simulink model "ANN_project"  (R2019b)
settings: Solver=ode45  StartTime=0.0  StopTime=0.6  RelTol=1e-3  EnableMultiTasking=on
libraries: powerlib x20
settings Model: Creator=Administrator  LastModifiedBy=Dell
settings DataIOCC: LimitDataPoints=on  SaveFormat=Array  SignalLoggingSaveFormat=ModelDataLogs  ReturnWorkspaceOutputs=off
settings OptimizationCC: ExpressionDepthLimit=2147483647  LifeSpan=inf
settings DebuggingCC: UnderspecifiedInitializationDetection=Classic  MergeDetectMultiDrivingBlocksExec=none  SolverPrmCheckMsg=warning  FcnCallInpInsideContextMsg=warning  StateNameClashWarn=warning  SFUnexpectedBacktrackingDiag=warning  SFNoUnconditionalDefaultTransitionDiag=warning  SFExecutionAtInitializationDiag=none  ArithmeticOperatorsInVariantConditions=warning
settings HardwareCC: ProdBitPerPointer=32  ProdBitPerSizeT=32  ProdBitPerPtrDiffT=32  ProdLargestAtomicFloat=None  ProdIntDivRoundTo=Undefined  ProdEndianess=Unspecified  ProdWordSize=32  ProdHWDeviceType=32-bit Generic
settings ModelReferenceCC: PropagateSignalLabelsOutOfModel=off
settings SFSimCC: SimUseLocalCustomCode=off  CustomCodeUndefinedFunction=UseInterfaceOnly
settings RTWCC: RTWUseLocalCustomCode=off
settings CodeAppCC: StateflowObjectComments=on
settings GRTTargetCC: TargetLangStandard=C89/C90 (ANSI)  GeneratePreprocessorConditionals=Disable all  CombineOutputUpdateFcns=off  GRTInterface=on
settings ConfigComp: CovMetricSettings=dw  CovHtmlReporting=on  CovSaveCumulativeToWorkspaceVar=on  CovSaveSingleToWorkspaceVar=on  CovExternalEMLEnable=off  CovSFcnEnable=off
settings SimscapeCC: SimscapeNormalizeSystem=off

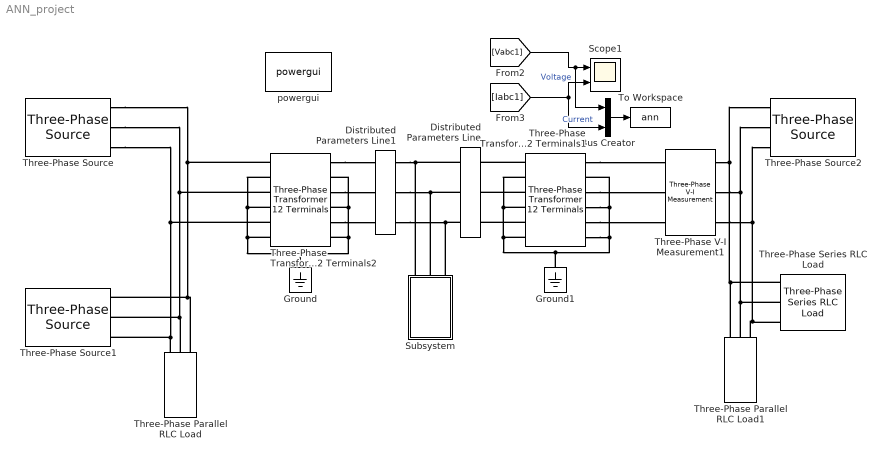
== system ANN_project ==
  Bus Creator : BusCreator  Inputs=2
  Distributed Parameters Line : powerlib/Elements/Distributed Parameters Line  Phases=3  Frequency=50  Resistance=[0.0132 0.132]  Inductance="[0.9337e-3  4.1264e-3]"  Capacitance=[12.74e-9 7.751e-9]  Length=33  x1=[-0.0002 1.11094093111666e-09 0 0;-0.00015 1.10646242430815e-09 15635.779124401 -78733.8101924462;-0.0001 1.10171091445278e-09 16870.5471169946 -78478.5008535489;-5e-05 1.09668757391454e-09 18101.1525545264 -78203.828118865]  x2=[-0.0002 1.10664892847414e-09 0 0;-0.00015 1.10142238341835e-09 15586.3909292958 -78738.689788468;-0.0001 1.0959240788704e-09 16821.2416601515 -78484.1556036391;-5e-05 1.09015537145464e-09 18051.9420013292 -78210.2566277985]  x3=[-0.0002 1.65913804517052e-12 0 0;-0.00015 1.64167462881892e-12 51.7591743809076 -286.446961708193;-0.0001 1.62380615381756e-12 56.2521023005705 -285.598625681592;-5e-05 1.60553702894529e-12 60.731150855709 -284.679822467609]  x4=[-0.0002 3.53794943184736e-13 0 0;-0.00015 3.43397446566386e-13 53.0400736803497 -296.594100248533;-0.0001 3.32915221766461e-13 57.6922279035049 -295.724392902892;-5e-05 3.22350855117083e-13 62.3301474326922 -294.781719988321]  x5=0.000186628717108595  V1=[2.547e-09 1.32e+05 1.32e+05;314.2 314.2 314.2;-0.1043 0.8095 -0.7613]  V2=[2.522e-09 1.32e+05 1.32e+05;314.2 314.2 314.2;-0.1193 0.8007 -0.7701]  I1=[2.615e-12 367.2 367.2;314.2 314.2 314.2;-0.5343 0.7771 -0.7937]  I2=[5.144e-12 607 607;314.2 314.2 314.2;-0.488 0.7934 -0.7774]  nHarmo=1  Measurements=None
      settings: SourceProductName=Simscape Electrical
  Distributed Parameters Line1 : powerlib/Elements/Distributed Parameters Line  Phases=3  Frequency=50  Resistance=[0.0132 0.132]  Inductance="[0.9337e-3  4.1264e-3]"  Capacitance=[12.74e-9 7.751e-9]  Length=33  x1=[-0.0002 1.06985997726373e-09 0 0;-0.00015 1.06563222080832e-09 15674.3204924214 -78626.6776409918;-0.0001 1.06114153554782e-09 16907.4009652819 -78370.7761372744;-5e-05 1.05638902949163e-09 18136.3097899451 -78095.5378172321]  x2=[-0.0002 1.11082671582699e-09 0 0;-0.00015 1.10637673817347e-09 15635.779124401 -78733.8101924462;-0.0001 1.10165377861486e-09 16870.5471169946 -78478.5008535489;-5e-05 1.09665900247079e-09 18101.1525545264 -78203.828118865]  x3=[-0.0002 1.50853045642763e-12 0 0;-0.00015 1.52159778925784e-12 41.4228708035809 -287.645866206956;-0.0001 1.53428969060172e-12 45.9359054607536 -286.959737874603;-5e-05 1.5466030289225e-12 50.4376061206075 -286.202806520801]  x4=[-0.0002 1.93791064768201e-12 0 0;-0.00015 1.91461187543894e-12 63.708177517745 -294.987739785213;-0.0001 1.89084070136455e-12 68.3337840298898 -293.950663320186;-5e-05 1.86660299064036e-12 72.9425302033257 -292.841058927463]  x5=0.000186628717108595  V1=[2.618e-09 1.319e+05 1.319e+05;314.2 314.2 314.2;-0.1003 0.8184 -0.7524]  V2=[2.549e-09 1.32e+05 1.32e+05;314.2 314.2 314.2;-0.1043 0.8095 -0.7613]  I1=[2.387e-12 367.3 367.3;314.2 314.2 314.2;0.1434 0.7414 -0.8294]  I2=[6.175e-12 607.4 607.4;314.2 314.2 314.2;-0.4569 0.8292 -0.7416]  nHarmo=1  Measurements=None
      settings: SourceProductName=Simscape Electrical
  Ground : powerlib/Elements/Ground  LConnTagsString=a
      settings: SourceProductName=Simscape Electrical
  Ground1 : powerlib/Elements/Ground  LConnTagsString=a
      settings: SourceProductName=Simscape Electrical
  Scope1 : Scope  NumInputPorts=2
  Subsystem : Subsystem
  Three-Phase Parallel RLC Load : powerlib/Elements/Three-Phase Parallel RLC Load  LConnTagsString=A|B|C  Configuration=Y (grounded)  NominalVoltage=1000  Vabc=[1e3 1e3 1e3]  Vabcp=[1e3 1e3 1e3]  NominalFrequency=60  UnbalancedPower=off  ActivePower=10e4  InductivePower=100  CapacitivePower=100  Pabc=[10e3 9e3 11e3]  QLabc=[100 90 110]  QCabc=[100 90 110]  Pabcp=[10e3 9e3 11e3]  QLabcp=[100 90 110]  QCabcp=[100 90 110]  Measurements=None  LoadType=constant Z
      settings: SourceProductName=Simscape Electrical
  Three-Phase Parallel RLC Load1 : powerlib/Elements/Three-Phase Parallel RLC Load  LConnTagsString=A|B|C  Configuration=Y (grounded)  NominalVoltage=1000  Vabc=[1e3 1e3 1e3]  Vabcp=[1e3 1e3 1e3]  NominalFrequency=60  UnbalancedPower=off  ActivePower=100  InductivePower=10  CapacitivePower=10  Pabc=[10e3 9e3 11e3]  QLabc=[100 90 110]  QCabc=[100 90 110]  Pabcp=[10e3 9e3 11e3]  QLabcp=[100 90 110]  QCabcp=[100 90 110]  Measurements=None  LoadType=constant Z
      settings: SourceProductName=Simscape Electrical
  Three-Phase Series RLC Load : powerlib/Elements/Three-Phase Series RLC Load  LConnTagsString=A|B|C  Configuration=Y (grounded)  NominalVoltage=11e3  Vabc=[1e3 1e3 1e3]  Vabcp=[1e3 1e3 1e3]  NominalFrequency=50  UnbalancedPower=off  ActivePower=10e6  InductivePower=100  CapacitivePower=0  Pabc=[10e3 9e3 11e3]  QLabc=[100 90 110]  QCabc=[100 90 110]  Pabcp=[10e3 9e3 11e3]  QLabcp=[100 90 110]  QCabcp=[100 90 110]  Measurements=None  LoadType=constant Z
      settings: SourceProductName=Simscape Electrical
  Three-Phase V-I Measurement1 : powerlib/Measurements/Three-Phase V-I Measurement  VoltageMeasurement=phase-to-phase  SetLabelV=on  LabelV=Vabc1  Vpu=off  VpuLL=on  CurrentMeasurement=yes  SetLabelI=on  LabelI=Iabc1  Ipu=off  Pbase=100e6  Vbase=11e3  OutputType=Complex  PhasorSimulation=off  PSBequivalent=0
      settings: SourceProductName=Simscape Electrical
  Three-Phase Source : powerlib/Electrical Sources/Three-Phase Source  InternalConnection=Yg  VoltagePhases=off  Voltage=11e3  PhaseAngle=0  Voltage_phases=[25e3 25e3 25e3]/sqrt(3)  PhaseAngles_phases=[0 -120 +120]  Frequency=50  NonIdealSource=on  SpecifyImpedance=off  Resistance=12  Inductance=16.58e-3  ShortCircuitLevel=50e6  BaseVoltage=11e3  XRratio=7  BusType=PV  Pref=50e6  Qref=0  Prefabc=[10e3, 10e3, 10e3]  Qrefabc=[0, 0, 0]  Qmin=-inf  Qmax=inf
      settings: SourceProductName=Simscape Electrical
  Three-Phase Source1 : powerlib/Electrical Sources/Three-Phase Source  InternalConnection=Yg  VoltagePhases=off  Voltage=11e3  PhaseAngle=0  Voltage_phases=[25e3 25e3 25e3]/sqrt(3)  PhaseAngles_phases=[0 -120 +120]  Frequency=50  NonIdealSource=on  SpecifyImpedance=off  Resistance=12  Inductance=16.58e-3  ShortCircuitLevel=50e6  BaseVoltage=11e3  XRratio=7  BusType=PV  Pref=50e6  Qref=0  Prefabc=[10e3, 10e3, 10e3]  Qrefabc=[0, 0, 0]  Qmin=-inf  Qmax=inf
      settings: SourceProductName=Simscape Electrical
  Three-Phase Source2 : powerlib/Electrical Sources/Three-Phase Source  InternalConnection=Yg  VoltagePhases=off  Voltage=11e3  PhaseAngle=0  Voltage_phases=[25e3 25e3 25e3]/sqrt(3)  PhaseAngles_phases=[0 -120 +120]  Frequency=50  NonIdealSource=on  SpecifyImpedance=off  Resistance=8.4  Inductance=16.58e-3  ShortCircuitLevel=20e6  BaseVoltage=11e3  XRratio=7  BusType=PV  Pref=20e6  Qref=0  Prefabc=[10e3, 10e3, 10e3]  Qrefabc=[0, 0, 0]  Qmin=-inf  Qmax=inf
      settings: SourceProductName=Simscape Electrical
  Three-Phase Transformer 12 Terminals1 : powerlib/Elements/Three-Phase Transformer 12 Terminals  RatedPower=[100e6 50]  Winding1="[ 132e3 0.002  0.05 ]"  Winding2=[ 11e3 0.002 0.05]  RmXm=[ 200 200 ]
      settings: SourceProductName=Simscape Electrical  SourceProductBaseCode=PS
  Three-Phase Transformer 12 Terminals2 : powerlib/Elements/Three-Phase Transformer 12 Terminals  RatedPower=[100e6 50]  Winding1="[ 11e3 0.002  0.05 ]"  Winding2=[ 132e3 0.002 0.05]  RmXm=[ 200 200 ]
      settings: SourceProductName=Simscape Electrical  SourceProductBaseCode=PS
  To Workspace : ToWorkspace  VariableName=ann  SaveFormat=Structure With Time  SampleTime=-1
  powergui : powerlib/powergui  Priority=1  SimulationMode=Discrete  SampleTime=50e-6  frequency=60  Iterations=50  frequencyindice=50  Pbase=100e6  ErrMax=1e-4  UnitsV=kV  UnitsW=MW  buscounter=0  FunctionMessages=off  echomessages=off  EnableUseOfTLC=off  CurrentSourceSwitches=off  DisableSnubberDevices=off  DisableRonSwitches=off  DisableVfSwitches=off  DisplayEquations=off  AutomaticDiscreteSolvers=off  SolverType=Tustin  Interpol=off  ExternalGateDelay=off  methode=off  Ts=0  x0status=blocks  SPID=off  SwTol=0  HookPort=off  NonlinearTolerance=1e-4  nMaxIteration=100  ContinueOnMaxIteration=off  RestoreLinks=warning  ResistiveCurrentMeasurement=off  Frange=[0:2:500]  Ylog=off  Xlog=on  ShowGrid=off  save=off  variable=ZData  structure=0  ZoomFFT=off  StartTime=0.0  cycles=1  DisplayStyle=1  fundamental=60  FreqAxis=off  MaxFrequency=1000  frequencyindicesteady=1  RmsSteady=1  display=off
      settings: SourceProductName=Simscape Electrical
  wires:
  [Vabc1] -> Bus Creator/1, Scope1/1  "Voltage"
  [Iabc1] -> Bus Creator/2, Scope1/2  "Current"
  Bus Creator/1 -> To Workspace/1
  connections:
  Distributed Parameters Line/LConn1 -- Subsystem/LConn1 -- Distributed Parameters Line1/RConn1
  Three-Phase Series RLC Load/LConn2 -- Three-Phase Parallel RLC Load1/LConn2 -- Three-Phase V-I Measurement1/RConn2 -- Three-Phase Source2/RConn2
  Distributed Parameters Line/LConn3 -- Distributed Parameters Line1/RConn3 -- Subsystem/LConn3
  Three-Phase Series RLC Load/LConn1 -- Three-Phase Parallel RLC Load1/LConn1 -- Three-Phase V-I Measurement1/RConn1 -- Three-Phase Source2/RConn1
  Distributed Parameters Line/LConn2 -- Subsystem/LConn2 -- Distributed Parameters Line1/RConn2
  Three-Phase Series RLC Load/LConn3 -- Three-Phase Parallel RLC Load1/LConn3 -- Three-Phase V-I Measurement1/RConn3 -- Three-Phase Source2/RConn3
  Three-Phase Transformer 12 Terminals1/LConn3 -- Distributed Parameters Line/RConn2
  Three-Phase Transformer 12 Terminals1/LConn1 -- Distributed Parameters Line/RConn1
  Three-Phase Transformer 12 Terminals1/LConn5 -- Distributed Parameters Line/RConn3
  Three-Phase Transformer 12 Terminals2/RConn1 -- Distributed Parameters Line1/LConn1
  Three-Phase Transformer 12 Terminals2/RConn3 -- Distributed Parameters Line1/LConn2
  Three-Phase Transformer 12 Terminals2/RConn5 -- Distributed Parameters Line1/LConn3
  Three-Phase Source/RConn2 -- Three-Phase Parallel RLC Load/LConn2 -- Three-Phase Source1/RConn2 -- Three-Phase Transformer 12 Terminals2/LConn3
  Three-Phase Source/RConn1 -- Three-Phase Parallel RLC Load/LConn3 -- Three-Phase Source1/RConn1 -- Three-Phase Transformer 12 Terminals2/LConn1
  Three-Phase Source/RConn3 -- Three-Phase Parallel RLC Load/LConn1 -- Three-Phase Source1/RConn3 -- Three-Phase Transformer 12 Terminals2/LConn5
  Three-Phase Transformer 12 Terminals1/RConn5 -- Three-Phase V-I Measurement1/LConn3
  Three-Phase Transformer 12 Terminals1/RConn3 -- Three-Phase V-I Measurement1/LConn2
  Three-Phase Transformer 12 Terminals1/RConn1 -- Three-Phase V-I Measurement1/LConn1
  Ground/LConn1 -- Three-Phase Transformer 12 Terminals2/LConn6 -- Three-Phase Transformer 12 Terminals2/LConn4 -- Three-Phase Transformer 12 Terminals2/LConn2 -- Three-Phase Transformer 12 Terminals2/RConn6 -- Three-Phase Transformer 12 Terminals2/RConn4 -- Three-Phase Transformer 12 Terminals2/RConn2
  Ground1/LConn1 -- Three-Phase Transformer 12 Terminals1/LConn2 -- Three-Phase Transformer 12 Terminals1/LConn4 -- Three-Phase Transformer 12 Terminals1/LConn6 -- Three-Phase Transformer 12 Terminals1/RConn6 -- Three-Phase Transformer 12 Terminals1/RConn4 -- Three-Phase Transformer 12 Terminals1/RConn2

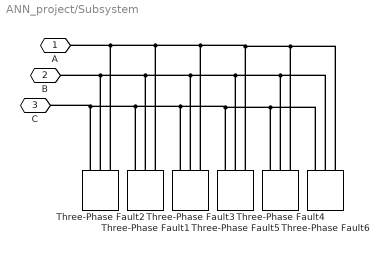
== system ANN_project/Subsystem ==
  Three-Phase Fault1 : powerlib/Elements/Three-Phase Fault  InitialStates=0  FaultA=on  FaultB=on  FaultC=off  GroundFault=on  SwitchTimes=[ 0.125 0.175]  External=off  SwitchStatus=NaN  FaultResistance=0.001  GroundResistance=0.001  SnubberResistance=1e6  SnubberCapacitance=inf  Measurements=None
      settings: SourceProductName=Simscape Electrical
  Three-Phase Fault2 : powerlib/Elements/Three-Phase Fault  InitialStates=0  FaultA=on  FaultB=off  FaultC=off  GroundFault=on  SwitchTimes=[ 0.025 0.075]  External=off  SwitchStatus=NaN  FaultResistance=0.001  GroundResistance=0.001  SnubberResistance=1e6  SnubberCapacitance=inf  Measurements=None
      settings: SourceProductName=Simscape Electrical
  Three-Phase Fault3 : powerlib/Elements/Three-Phase Fault  InitialStates=0  FaultA=off  FaultB=on  FaultC=on  GroundFault=off  SwitchTimes=[ 0.225 0.275]  External=off  SwitchStatus=NaN  FaultResistance=0.001  GroundResistance=0.001  SnubberResistance=1e6  SnubberCapacitance=inf  Measurements=None
      settings: SourceProductName=Simscape Electrical
  Three-Phase Fault4 : powerlib/Elements/Three-Phase Fault  InitialStates=0  FaultA=on  FaultB=on  FaultC=on  GroundFault=on  SwitchTimes=[ 0.425 0.475]  External=off  SwitchStatus=NaN  FaultResistance=0.001  GroundResistance=0.001  SnubberResistance=1e6  SnubberCapacitance=inf  Measurements=None
      settings: SourceProductName=Simscape Electrical
  Three-Phase Fault5 : powerlib/Elements/Three-Phase Fault  InitialStates=0  FaultA=on  FaultB=on  FaultC=on  GroundFault=off  SwitchTimes=[ 0.325 0.375]  External=off  SwitchStatus=NaN  FaultResistance=0.001  GroundResistance=0.001  SnubberResistance=1e6  SnubberCapacitance=inf  Measurements=None
      settings: SourceProductName=Simscape Electrical
  Three-Phase Fault6 : powerlib/Elements/Three-Phase Fault  InitialStates=0  FaultA=off  FaultB=off  FaultC=off  GroundFault=off  SwitchTimes=[ 0.525 0.575]  External=off  SwitchStatus=NaN  FaultResistance=0.001  GroundResistance=0.001  SnubberResistance=1e6  SnubberCapacitance=inf  Measurements=None
      settings: SourceProductName=Simscape Electrical
  A : PMIOPort  Side=Left
  B : PMIOPort  Port=2  Side=Left
  C : PMIOPort  Port=3  Side=Left
  connections:
  Three-Phase Fault2/LConn2 -- Three-Phase Fault6/LConn2 -- Three-Phase Fault4/LConn2 -- Three-Phase Fault5/LConn2 -- Three-Phase Fault3/LConn2 -- Three-Phase Fault1/LConn2 -- B/RConn1
  Three-Phase Fault2/LConn3 -- Three-Phase Fault6/LConn3 -- Three-Phase Fault4/LConn3 -- Three-Phase Fault5/LConn3 -- Three-Phase Fault3/LConn3 -- Three-Phase Fault1/LConn3 -- C/RConn1
  Three-Phase Fault2/LConn1 -- Three-Phase Fault6/LConn1 -- Three-Phase Fault4/LConn1 -- Three-Phase Fault5/LConn1 -- Three-Phase Fault3/LConn1 -- Three-Phase Fault1/LConn1 -- A/RConn1
